simulink model "ANTIGOcontrolador"  (R2021a)
settings: Solver=ode23t  StartTime=0.0  StopTime=60  MaxStep=1e-3  RelTol=1e-3
values from neighbouring files (symbols this model uses):
  AL = double(subs(A_par))    [ANTImodeloMATEMATICOFINAL.m]
  BL = double(subs(B_par))    [ANTImodeloMATEMATICOFINAL.m]
  Blo = 8.18575752786119e-06    (= 8.18575752786e-06)    [ANTImodeloMATEMATICOFINAL.m]
  Bmo = 2.02156082362446e-07    (= 2.02156082362e-07)    [ANTImodeloMATEMATICOFINAL.m]
  CL = double(subs(C_par))    [ANTImodeloMATEMATICOFINAL.m]
  DL = double(subs(D_par))    [ANTImodeloMATEMATICOFINAL.m]
  do = 0.06862-0.021    (= 0.04762)    [ANTImodeloMATEMATICOFINAL.m]
  go = 9.81    [ANTImodeloMATEMATICOFINAL.m]
  Jlo = 0.00100697016255642    (= 0.00100697016256)    [ANTImodeloMATEMATICOFINAL.m]
  Jmo = 2.08549279330578e-07    (= 2.08549279331e-07)    [ANTImodeloMATEMATICOFINAL.m]
  Kes = K(:,1:n)    [ANTImodeloMATEMATICOFINAL.m]
  Ki = -K(:,n+1:end)    [ANTImodeloMATEMATICOFINAL.m]
  Kio = 0.00119530882984502    (= 0.00119530882985)    [ANTImodeloMATEMATICOFINAL.m]
  Kvo = 0.0035694528924319    (= 0.00356945289243)    [ANTImodeloMATEMATICOFINAL.m]
  Lo = 0.667669785204658    (= 0.667669785205)    [ANTImodeloMATEMATICOFINAL.m]
  mo = 0.17244    [ANTImodeloMATEMATICOFINAL.m]
  no = 120    [ANTImodeloMATEMATICOFINAL.m]
  Ro = 5.15610211779038    (= 5.15610211779)    [ANTImodeloMATEMATICOFINAL.m]
  Tm = 0.03    [ANTImodeloMATEMATICOFINAL.m]
  Vin0 = Ro*X10    (= 0)    [ANTImodeloMATEMATICOFINAL.m]
  X10 = 0    [ANTImodeloMATEMATICOFINAL.m]
  X20 = 0    [ANTImodeloMATEMATICOFINAL.m]
  X30 = 0    [ANTImodeloMATEMATICOFINAL.m]
libraries: cstblocks x6, slpidlib x4
(part 2 of 2)

== matlab function ANTIGOcontrolador/Seg. Estados/Subsystem2/MATLAB Function ==
  data: x input; PWM input; dx output; parametros input
function dx = fcn(x,PWM,parametros)

%ESTADOS
x1 = x(1);
x2 = x(2);

%Parametros
R = parametros(1);
L = parametros(2);
Ki = parametros(3);
Kv = parametros(4);
Jm = parametros(5);
Jl = parametros(6);
Bm = parametros(7);
Bl = parametros(8);
n = parametros(9);
g = parametros(10);
d = parametros(11);
m = parametros(12);

%EXPRESIONES
f1 = x2; %d0l/dt = Wl
f2= ((Ki*(((7*PWM/100)-(Kv*x2*n)/R))*n)-x2*(Bm*n^2+Bl)-(m*g*d*sin(x1)))/(Jl+Jm*n^2);

dx = [f1; f2];

== matlab function ANTIGOcontrolador/Estados Discreto/Subsystem1/MATLAB Function ==
  data: x input; PWM input; dx output; parametros input
function dx = fcn(x,PWM,parametros)

%ESTADOS
x1 = x(1);
x2 = x(2);

%Parametros
R = parametros(1);
L = parametros(2);
Ki = parametros(3);
Kv = parametros(4);
Jm = parametros(5);
Jl = parametros(6);
Bm = parametros(7);
Bl = parametros(8);
n = parametros(9);
g = parametros(10);
d = parametros(11);
m = parametros(12);

%EXPRESIONES
f1 = x2; %d0l/dt = Wl
f2= ((Ki*(((7*PWM/100)-(Kv*x2*n)/R))*n)-x2*(Bm*n^2+Bl)-(m*g*d*sin(x1)))/(Jl+Jm*n^2);

dx = [f1; f2];

== matlab function ANTIGOcontrolador/PID 1 DOF /Subsystem/MATLAB Function ==
  data: x input; PWM input; dx output; parametros input
function dx = fcn(x,PWM,parametros)

%ESTADOS
x1 = x(1);
x2 = x(2);
x3 = x(3);

%Parametros
R = parametros(1);
L = parametros(2);
Ki = parametros(3);
Kv = parametros(4);
Jm = parametros(5);
Jl = parametros(6);
Bm = parametros(7);
Bl = parametros(8);
n = parametros(9);
g = parametros(10);
d = parametros(11);
m = parametros(12);

%EXPRESIONES
% Jt = Jm*n^2 +Jl;
% f1 = (1/L)*(((7*PWM)/100) - R*x1 - Kv*x2*n);
% f2 = (1/Jt)*(Ki*x1*n - (Bm*n^2 + Bl)*x2 - m*g*d*sin(x3));
% f3 = x2;

% MODELO 2 ESTADOS I TL WL  SALIDA TL WL
f1 = (((7*PWM)/100)-Kv*x3*n-R*x1)/(L); %di/dt
f2 = x3; %d0l/dt = Wl
f3 = ((Ki*x1*n)-x3*(Bm*n^2+Bl)-(m*g*d*sin(x2)))/(Jl+Jm*n^2);  %dwl/dt 

dx = [f1; f2; f3];

== matlab function ANTIGOcontrolador/PID 1 DOF Discreto/Subsystem/MATLAB Function ==
  data: x input; PWM input; dx output; parametros input
function dx = fcn(x,PWM,parametros)

%ESTADOS
x1 = x(1);
x2 = x(2);
x3 = x(3);

%Parametros
R = parametros(1);
L = parametros(2);
Ki = parametros(3);
Kv = parametros(4);
Jm = parametros(5);
Jl = parametros(6);
Bm = parametros(7);
Bl = parametros(8);
n = parametros(9);
g = parametros(10);
d = parametros(11);
m = parametros(12);
Cm = 0.005;

if x3 > 0
    Ft = Bm*sign(x3) - Cm*x3;
elseif x3 <0
        Ft = Bm*sign(x3) + Cm*x3;
else
    Ft = 0;
end



if abs(PWM)<20
    x3 = 0;
end



% MODELO 2 ESTADOS I TL WL  SALIDA TL WL
f1 = (((7*PWM)/100)-Kv*x3*n-R*x1)/(L); %di/dt
f2 = x3; %d0l/dt = Wl
f3 = ((Ki*x1*n)-x3*(Bm*n^2+Bl)-(m*g*d*sin(x2)) - Ft)/(Jl+Jm*n^2);  %dwl/dt 

if abs(PWM)<20
    f3= 0;
end

dx = [f1; f2; f3];



% function dx = fcn(x,PWM,parametros)
% 
% %ESTADOS
% x1 = x(1);
% x2 = x(2);
% x3 = x(3);
% 
% %Parametros
% R = parametros(1);
% L = parametros(2);
% Ki = parametros(3);
% Kv = parametros(4);
% Jm = parametros(5);
% Jl = parametros(6);
% Bm = parametros(7);
% Bl = parametros(8);
% n = parametros(9);
% g = parametros(10);
% d = parametros(11);
% m = parametros(12);
% V = 3.94;
% % Incluir los parametros añadidos
% % Incluir la diiferencia de PWM que se debe aplciar al motor para que este
% % cambie de posicion EN LAZO ABIERTO
% difPWM = 30;
% % Incluir la velocidad minima que puede mantener el motor
% velMinima = 0.05;
% 
% if abs(PWM)<30
%     x3 = 0;
% end
% 
% Fs = ((difPWM*V/100)/R)*(Ki+Kv); % Friccion estatica
% Fc = Fs/8; % Friccion de Coulumb
% % Determinar la friccion TOTAL que se aplica al modelo
% % Torque externo
% Tex = - m*g*d*sin(x2) + (Ki+Kv)*x1;
% % Si la velocidad es menor a la velocidad minima entonces se aplica
% % FRICCION ESTATICA
% if(abs(x3) <= velMinima)
% if(abs(Tex) <= (Fs))
% % la friccion es igual al torque externo
% Ft = -Tex ;
% else
% % la friccion es igual a la suma de las fricciones
% Ft = -(Fs)*sign(Tex);
% end
% % Si la velocidad es mayor a la velocidad minima entonces se aplica
% % FRICCION COULUMB (unicamente)
% else
% Ft = -Fc*sign(x3);
% end
% 
% 
% 
% 
% 
% 
% % MODELO 2 ESTADOS I TL WL  SALIDA TL WL
% % MODELO 2 ESTADOS I TL WL  SALIDA TL WL
% f1 = (((7*PWM)/100)-Kv*x3*n-R*x1)/(L); %di/dt
% f2 = x3; %d0l/dt = Wl
% f3 = ((Ki*x1*n)-x3*(Bm*n^2+Bl)-(m*g*d*sin(x2)) - Ft)/(Jl+Jm*n^2);  %dwl/dt 
% 
% if abs(PWM)<30
%     f3 = 0;
% end
% 
% dx = [f1; f2; f3];

== matlab function ANTIGOcontrolador/Estados Discreto/MATLAB Function ==
  data: Sp input; us output; X_est input; Con_ini input; Con_out output
function [us,Con_out] = fcn(Sp,X_est,Con_ini)

umax = 100;
umin = -100;
kaw = zeros(1);
CL = [1, 0]
Ki = [13.038404810405284];
Kes = [8.39272964861829,6.19627625077861];

Vk_1 = Con_ini(1);
dif_act = Con_ini(2);

Tm = 0.03;
Kid = Ki*Tm;

Pv = CL*X_est;
en = Sp - Pv;
Vk = en + Vk_1 + kaw*dif_act;
un = Kid*Vk - Kes*X_est;
us = un;

Vk_1 = Vk;

if un>umax
    us = umax;
end
if un<umin
    us = umin;
end

dif_act = us - un;
Con_out = [Vk_1; dif_act];
